simulink library "sm_excv_underc_lib"  (R2023b)
settings: Solver=VariableStepAuto  StartTime=0.0  StopTime=10.0  RelTol=1e-3
undefined symbols (not defined in the file): Excv, L1, L2, L3, L4, L5, L6, L7, L8, L9, P1, P2, P3, P4, P5, P6, P7, P8, P9, shoe_w, X, Y, Z
libraries: sm_tracked_vehicle_lib x70, sm_lib x54, nesl_utility x32, sm_excv_scene_lib x9, fl_lib x8, sm_excv_frame_lib x4
(part 4 of 5)

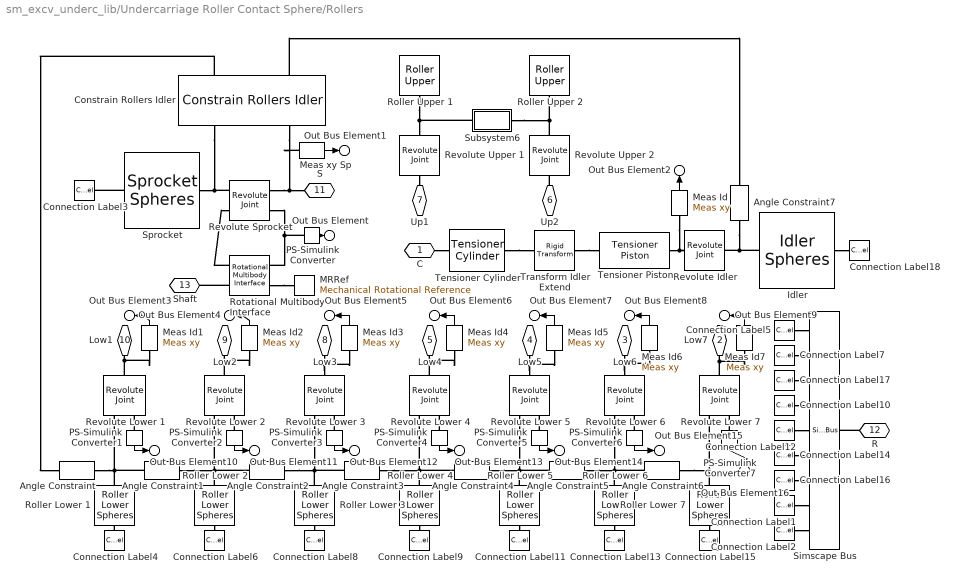
== system sm_excv_underc_lib/Undercarriage Roller Contact Sphere/Rollers ==
  Angle Constraint{,1..7} (8 alike) : sm_tracked_vehicle_lib/Angle Constraint  SystemSampleTime=-1  VariantActivationTime=update diagram  AllowFlexibleInterface=on  Latency=0  AutoFrameSizeCalculation=off
  Connection Label1 : ConnectionLabel  Label=Spr
  Connection Label10 : ConnectionLabel  Label=L4
  Connection Label11 : ConnectionLabel  Label=L5
  Connection Label12 : ConnectionLabel  Label=L5
  Connection Label13 : ConnectionLabel  Label=L6
  Connection Label14 : ConnectionLabel  Label=L6
  Connection Label15 : ConnectionLabel  Label=L7
  Connection Label16 : ConnectionLabel  Label=L7
  Connection Label17 : ConnectionLabel  Label=L3
  Connection Label18 : ConnectionLabel  Label=Idl
  Connection Label2 : ConnectionLabel  Label=Idl
  Connection Label3 : ConnectionLabel  Label=Spr
  Connection Label4 : ConnectionLabel  Label=L1
  Connection Label5 : ConnectionLabel  Label=L1
  Connection Label6 : ConnectionLabel  Label=L2
  Connection Label7 : ConnectionLabel  Label=L2
  Connection Label8 : ConnectionLabel  Label=L3
  Connection Label9 : ConnectionLabel  Label=L4
  Constrain Rollers Idler : sm_tracked_vehicle_lib/Constrain Rollers Idler  sprk_rolling_rad=sprk_rolling_rad  roller_lower_rolling_rad=roller_lower_rolling_rad  idler_rolling_rad=idler_rolling_rad
  Idler : sm_tracked_vehicle_lib/Idler Spheres  idler_rad=idler_rad  idler_len=idler_len  idler_rho=idler_rho  idler_clr=idler_clr  idler_opc=idler_opc  idler_rolling_rad=idler_rolling_rad  idler_contact_geo_width=shoe_w  idler_contact_geo_clr=idler_contact_geo_clr  idler_contact_geo_opc=idler_contact_geo_opc
  MRRef : fl_lib/Mechanical/Rotational Elements/Mechanical Rotational Reference
  Meas Id{,1..7} (8 alike) : sm_excv_scene_lib/Meas xy  whl_offset=Excv.Shoe.w
  Meas xy Sp : sm_excv_scene_lib/Meas xy  whl_offset=Excv.Shoe.w
  PS-Simulink Converter{,1..7} (8 alike) : nesl_utility/PS-Simulink Converter  PhysicalDomain=network_engine_domain  SubClassName=ps_output  LeftPortType=input  RightPortType=output  PseudoPeriodic=off  Frequencies=[]  VectorFormat=inherit  Unit=inherit  AffineConversion=off
  Revolute Idler : sm_lib/Joints/Revolute Joint  JointMode=Normal  SenseConstraintForce=off  SenseConstraintForceX=off  SenseConstraintForceY=off  SenseConstraintForceZ=off  SenseConstraintTorque=off  SenseConstraintTorqueX=off  SenseConstraintTorqueY=off  SenseConstraintTorqueZ=off  SenseTotalForce=off  SenseTotalForceX=off  SenseTotalForceY=off  SenseTotalForceZ=off  SenseTotalTorque=off  SenseTotalTorqueX=off  SenseTotalTorqueY=off  SenseTotalTorqueZ=off  CompositeWrenchDir=FollowerOnBase  CompositeWrenchFrame=BaseFrame  EquilibriumPosition=0  EquilibriumPositionUnits=rad  SpringStiffness=0  SpringStiffnessUnits=N*m/rad  DampingCoefficient=0  DampingCoefficientUnits=N*m/(rad/s)  TorqueActuationMode=NoTorque  MotionActuationMode=ComputedMotion  SensePosition=off  SenseVelocity=off  SenseAcceleration=off  SenseTorqueForce=off  SenseLowerLimitTorqueForce=off  SenseUpperLimitTorqueForce=off  LowerLimitSpecify=off  LowerLimitBound=-90  LowerLimitBoundUnits=deg  LowerLimitStiffness=1e4  LowerLimitStiffnessUnits=N*m/deg  LowerLimitDamping=10  LowerLimitDampingUnits=N*m/(deg/s)  LowerLimitTransitionRegionWidth=0.1  LowerLimitTransitionRegionWidthUnits=deg  UpperLimitSpecify=off  UpperLimitBound=90  UpperLimitBoundUnits=deg  UpperLimitStiffness=1e4  UpperLimitStiffnessUnits=N*m/deg  UpperLimitDamping=10  UpperLimitDampingUnits=N*m/(deg/s)  UpperLimitTransitionRegionWidth=0.1  UpperLimitTransitionRegionWidthUnits=deg  PositionTargetSpecify=off  PositionTargetPriority=Low  PositionTargetValue=0  PositionTargetValueUnits=deg  VelocityTargetSpecify=off  VelocityTargetPriority=High  VelocityTargetValue=0  VelocityTargetValueUnits=deg/s
  Revolute Lower {1..7} (7 alike) : sm_lib/Joints/Revolute Joint  JointMode=Normal  SenseConstraintForce=off  SenseConstraintForceX=off  SenseConstraintForceY=off  SenseConstraintForceZ=off  SenseConstraintTorque=off  SenseConstraintTorqueX=off  SenseConstraintTorqueY=off  SenseConstraintTorqueZ=off  SenseTotalForce=off  SenseTotalForceX=off  SenseTotalForceY=off  SenseTotalForceZ=off  SenseTotalTorque=off  SenseTotalTorqueX=off  SenseTotalTorqueY=off  SenseTotalTorqueZ=off  CompositeWrenchDir=FollowerOnBase  CompositeWrenchFrame=BaseFrame  EquilibriumPosition=0  EquilibriumPositionUnits=rad  SpringStiffness=0  SpringStiffnessUnits=N*m/rad  DampingCoefficient=0  DampingCoefficientUnits=N*m/(rad/s)  TorqueActuationMode=NoTorque  MotionActuationMode=ComputedMotion  SensePosition=off  SenseVelocity=off  SenseAcceleration=off  SenseTorqueForce=on  SenseLowerLimitTorqueForce=off  SenseUpperLimitTorqueForce=off  LowerLimitSpecify=off  LowerLimitBound=-90  LowerLimitBoundUnits=deg  LowerLimitStiffness=1e4  LowerLimitStiffnessUnits=N*m/deg  LowerLimitDamping=10  LowerLimitDampingUnits=N*m/(deg/s)  LowerLimitTransitionRegionWidth=0.1  LowerLimitTransitionRegionWidthUnits=deg  UpperLimitSpecify=off  UpperLimitBound=90  UpperLimitBoundUnits=deg  UpperLimitStiffness=1e4  UpperLimitStiffnessUnits=N*m/deg  UpperLimitDamping=10  UpperLimitDampingUnits=N*m/(deg/s)  UpperLimitTransitionRegionWidth=0.1  UpperLimitTransitionRegionWidthUnits=deg  PositionTargetSpecify=off  PositionTargetPriority=Low  PositionTargetValue=0  PositionTargetValueUnits=deg  VelocityTargetSpecify=off  VelocityTargetPriority=High  VelocityTargetValue=0  VelocityTargetValueUnits=deg/s
  Revolute Sprocket : sm_lib/Joints/Revolute Joint  JointMode=Normal  SenseConstraintForce=off  SenseConstraintForceX=off  SenseConstraintForceY=off  SenseConstraintForceZ=off  SenseConstraintTorque=off  SenseConstraintTorqueX=off  SenseConstraintTorqueY=off  SenseConstraintTorqueZ=off  SenseTotalForce=off  SenseTotalForceX=off  SenseTotalForceY=off  SenseTotalForceZ=off  SenseTotalTorque=off  SenseTotalTorqueX=off  SenseTotalTorqueY=off  SenseTotalTorqueZ=off  CompositeWrenchDir=FollowerOnBase  CompositeWrenchFrame=BaseFrame  EquilibriumPosition=0  EquilibriumPositionUnits=rad  SpringStiffness=0  SpringStiffnessUnits=N*m/rad  DampingCoefficient=0  DampingCoefficientUnits=N*m/(rad/s)  TorqueActuationMode=InputTorque  MotionActuationMode=ComputedMotion  SensePosition=off  SenseVelocity=on  SenseAcceleration=off  SenseTorqueForce=off  SenseLowerLimitTorqueForce=off  SenseUpperLimitTorqueForce=off  LowerLimitSpecify=off  LowerLimitBound=-90  LowerLimitBoundUnits=deg  LowerLimitStiffness=1e4  LowerLimitStiffnessUnits=N*m/deg  LowerLimitDamping=10  LowerLimitDampingUnits=N*m/(deg/s)  LowerLimitTransitionRegionWidth=0.1  LowerLimitTransitionRegionWidthUnits=deg  UpperLimitSpecify=off  UpperLimitBound=90  UpperLimitBoundUnits=deg  UpperLimitStiffness=1e4  UpperLimitStiffnessUnits=N*m/deg  UpperLimitDamping=10  UpperLimitDampingUnits=N*m/(deg/s)  UpperLimitTransitionRegionWidth=0.1  UpperLimitTransitionRegionWidthUnits=deg  PositionTargetSpecify=off  PositionTargetPriority=Low  PositionTargetValue=0  PositionTargetValueUnits=deg  VelocityTargetSpecify=off  VelocityTargetPriority=High  VelocityTargetValue=0  VelocityTargetValueUnits=deg/s
  Revolute Upper 1 : sm_lib/Joints/Revolute Joint  JointMode=Normal  SenseConstraintForce=off  SenseConstraintForceX=off  SenseConstraintForceY=off  SenseConstraintForceZ=off  SenseConstraintTorque=off  SenseConstraintTorqueX=off  SenseConstraintTorqueY=off  SenseConstraintTorqueZ=off  SenseTotalForce=off  SenseTotalForceX=off  SenseTotalForceY=off  SenseTotalForceZ=off  SenseTotalTorque=off  SenseTotalTorqueX=off  SenseTotalTorqueY=off  SenseTotalTorqueZ=off  CompositeWrenchDir=FollowerOnBase  CompositeWrenchFrame=BaseFrame  EquilibriumPosition=0  EquilibriumPositionUnits=rad  SpringStiffness=0  SpringStiffnessUnits=N*m/rad  DampingCoefficient=0  DampingCoefficientUnits=N*m/(rad/s)  TorqueActuationMode=NoTorque  MotionActuationMode=ComputedMotion  SensePosition=off  SenseVelocity=off  SenseAcceleration=off  SenseTorqueForce=off  SenseLowerLimitTorqueForce=off  SenseUpperLimitTorqueForce=off  LowerLimitSpecify=off  LowerLimitBound=-90  LowerLimitBoundUnits=deg  LowerLimitStiffness=1e4  LowerLimitStiffnessUnits=N*m/deg  LowerLimitDamping=10  LowerLimitDampingUnits=N*m/(deg/s)  LowerLimitTransitionRegionWidth=0.1  LowerLimitTransitionRegionWidthUnits=deg  UpperLimitSpecify=off  UpperLimitBound=90  UpperLimitBoundUnits=deg  UpperLimitStiffness=1e4  UpperLimitStiffnessUnits=N*m/deg  UpperLimitDamping=10  UpperLimitDampingUnits=N*m/(deg/s)  UpperLimitTransitionRegionWidth=0.1  UpperLimitTransitionRegionWidthUnits=deg  PositionTargetSpecify=off  PositionTargetPriority=Low  PositionTargetValue=0  PositionTargetValueUnits=deg  VelocityTargetSpecify=off  VelocityTargetPriority=High  VelocityTargetValue=0  VelocityTargetValueUnits=deg/s
  Revolute Upper 2 : sm_lib/Joints/Revolute Joint  JointMode=Normal  SenseConstraintForce=off  SenseConstraintForceX=off  SenseConstraintForceY=off  SenseConstraintForceZ=off  SenseConstraintTorque=off  SenseConstraintTorqueX=off  SenseConstraintTorqueY=off  SenseConstraintTorqueZ=off  SenseTotalForce=off  SenseTotalForceX=off  SenseTotalForceY=off  SenseTotalForceZ=off  SenseTotalTorque=off  SenseTotalTorqueX=off  SenseTotalTorqueY=off  SenseTotalTorqueZ=off  CompositeWrenchDir=FollowerOnBase  CompositeWrenchFrame=BaseFrame  EquilibriumPosition=0  EquilibriumPositionUnits=rad  SpringStiffness=0  SpringStiffnessUnits=N*m/rad  DampingCoefficient=0  DampingCoefficientUnits=N*m/(rad/s)  TorqueActuationMode=NoTorque  MotionActuationMode=ComputedMotion  SensePosition=off  SenseVelocity=off  SenseAcceleration=off  SenseTorqueForce=off  SenseLowerLimitTorqueForce=off  SenseUpperLimitTorqueForce=off  LowerLimitSpecify=off  LowerLimitBound=-90  LowerLimitBoundUnits=deg  LowerLimitStiffness=1e4  LowerLimitStiffnessUnits=N*m/deg  LowerLimitDamping=10  LowerLimitDampingUnits=N*m/(deg/s)  LowerLimitTransitionRegionWidth=0.1  LowerLimitTransitionRegionWidthUnits=deg  UpperLimitSpecify=off  UpperLimitBound=90  UpperLimitBoundUnits=deg  UpperLimitStiffness=1e4  UpperLimitStiffnessUnits=N*m/deg  UpperLimitDamping=10  UpperLimitDampingUnits=N*m/(deg/s)  UpperLimitTransitionRegionWidth=0.1  UpperLimitTransitionRegionWidthUnits=deg  PositionTargetSpecify=off  PositionTargetPriority=Low  PositionTargetValue=0  PositionTargetValueUnits=deg  VelocityTargetSpecify=off  VelocityTargetPriority=High  VelocityTargetValue=0  VelocityTargetValueUnits=deg/s
  Roller Lower {1..7} (7 alike) : sm_tracked_vehicle_lib/Roller Lower Spheres  roller_lower_rad=roller_lower_rad  roller_lower_len=roller_lower_len  roller_lower_rho=roller_lower_rho  roller_lower_clr=roller_lower_clr  roller_lower_opc=roller_lower_opc  roller_lower_rolling_rad=roller_lower_rolling_rad  roller_lower_contgeo_width=shoe_w  roller_lower_contgeo_clr=roller_lower_contgeo_clr  roller_lower_contgeo_opc=roller_lower_contgeo_opc
      settings: LibrarySourceBlock=sm_chain_drive_lib/Pulley_Bot
  Roller Upper 1 : sm_tracked_vehicle_lib/Roller Upper  roller_upper_rad=roller_upper_rad  roller_upper_len=roller_upper_len  roller_upper_rho=roller_upper_rho  roller_upper_clr=roller_upper_clr  roller_upper_opc=roller_upper_opc  roller_upper_contgeo_clr=roller_upper_contgeo_clr  roller_upper_contgeo_opc=roller_upper_contgeo_opc
      settings: LibrarySourceBlock=sm_chain_drive_lib/Pulley_Top
  Roller Upper 2 : sm_tracked_vehicle_lib/Roller Upper  roller_upper_rad=roller_upper_rad  roller_upper_len=roller_upper_len  roller_upper_rho=roller_upper_rho  roller_upper_clr=roller_upper_clr  roller_upper_opc=roller_upper_opc  roller_upper_contgeo_clr=roller_upper_contgeo_clr  roller_upper_contgeo_opc=roller_upper_contgeo_opc
      settings: LibrarySourceBlock=sm_chain_drive_lib/Pulley_Top
  Rotational Multibody Interface : fl_lib/Mechanical/Multibody Interfaces/Rotational Multibody Interface
  Simscape Bus : SimscapeBus  HierarchyStrings=L1;L2;L3;L4;L5;L6;L7;L8;L9
  Sprocket : sm_tracked_vehicle_lib/Sprocket Spheres  sprk_xc=sprk_xc  sprk_len=sprk_len  sprk_rho=sprk_rho  sprk_clr=sprk_clr  sprk_opc=sprk_opc  sprk_rolling_rad=sprk_rolling_rad  sprk_contact_geo_w=shoe_w  sprk_contact_geo_clr=sprk_contact_geo_clr  sprk_contact_geo_opc=sprk_contact_geo_opc
  Subsystem6 : Subsystem
  Tensioner Cylinder : sm_tracked_vehicle_lib/Tensioner Cylinder  cyl_rad=tensioner_cyl_rad  cyl_len=tensioner_cyl_len  cyl_rho=tensioner_cyl_rho  cyl_clr=tensioner_cyl_clr  cyl_opc=tensioner_cyl_opc
      settings: LibrarySourceBlock=sm_chain_drive_lib/Idler_Housing
  Tensioner Piston : sm_tracked_vehicle_lib/Tensioner Piston  pist_rad=tensioner_pist_rad  pist_len=tensioner_pist_len  pist_rho=tensioner_pist_rho  pist_clr=tensioner_pist_clr  pist_opc=tensioner_pist_opc  br_height=tensioner_br_height  br_length=tensioner_br_length  br_width=tensioner_br_width  br_rho=tensioner_br_rho  br_thk=tensioner_br_thk  br_clr=tensioner_br_clr  br_opc=tensioner_br_opc
      settings: LibrarySourceBlock=sm_chain_drive_lib/ldler_Damper
  Transform Idler Extend : sm_lib/Frames and Transforms/Rigid Transform  TranslationMethod=StandardAxis  TranslationStandardOffset=idler_max_ext  TranslationStandardOffsetUnits=m  TranslationStandardAxis=+Z  TranslationCartesianOffset=[0 0 0]  TranslationCartesianOffsetUnits=m  TranslationROffset=0  TranslationROffsetUnits=m  TranslationZOffset=0  TranslationZOffsetUnits=m  TranslationThetaOffset=0  TranslationThetaOffsetUnits=deg  RotationMethod=None  RotationAngleUnits=deg  RotationStandardAxis=+Z  RotationAngle=0.1  RotationArbitraryAxis=[0 0 1]  FollAlignAxisA=+X  BaseAlignAxisA=+Y  FollAlignAxisB=+Y  BaseAlignAxisB=+Z  RotationSequenceAxes=FollowerAxes  RotationSequence=XYX  RotationSequenceAngles=[0 0 0]  RotationSequenceAnglesUnits=deg  RotationMatrix=[1 0 0; 0 1 0; 0 0 1]  Quaternion=[1 0 0 0]
  C : PMIOPort  Side=Left
  Low7 : PMIOPort  Port=2  Side=Left
  Low6 : PMIOPort  Port=3  Side=Left
  Low5 : PMIOPort  Port=4  Side=Left
  Low4 : PMIOPort  Port=5  Side=Left
  Up2 : PMIOPort  Port=6  Side=Left
  Up1 : PMIOPort  Port=7  Side=Left
  Low3 : PMIOPort  Port=8  Side=Left
  Low2 : PMIOPort  Port=9  Side=Left
  Low1 : PMIOPort  Port=10  Side=Left
  S : PMIOPort  Port=11  Side=Left
  R : PMIOPort  Port=12  Side=Right
  Shaft : PMIOPort  Port=13  Side=Right
  Out Bus Element : Outport  PortName=m  Element=tSprk
  Out Bus Element1 : Outport  PortName=m  Element=Sp
  Out Bus Element2 : Outport  PortName=m  Element=Id
  Out Bus Element3 : Outport  PortName=m  Element=LR1
  Out Bus Element4 : Outport  PortName=m  Element=LR2
  Out Bus Element5 : Outport  PortName=m  Element=LR3
  Out Bus Element6 : Outport  PortName=m  Element=LR4
  Out Bus Element7 : Outport  PortName=m  Element=LR5
  Out Bus Element8 : Outport  PortName=m  Element=LR6
  Out Bus Element9 : Outport  PortName=m  Element=LR7
  Out Bus Element10 : Outport  PortName=m  Element=RL1
  Out Bus Element11 : Outport  PortName=m  Element=RL2
  Out Bus Element12 : Outport  PortName=m  Element=RL3
  Out Bus Element13 : Outport  PortName=m  Element=RL4
  Out Bus Element14 : Outport  PortName=m  Element=RL5
  Out Bus Element15 : Outport  PortName=m  Element=RL6
  Out Bus Element16 : Outport  PortName=m  Element=RL7
  wires:
  PS-Simulink Converter/1 -> Out Bus Element/1
  Meas xy Sp/1 -> Out Bus Element1/1
  Meas Id/1 -> Out Bus Element2/1
  Meas Id1/1 -> Out Bus Element3/1
  Meas Id2/1 -> Out Bus Element4/1
  Meas Id3/1 -> Out Bus Element5/1
  Meas Id4/1 -> Out Bus Element6/1
  Meas Id5/1 -> Out Bus Element7/1
  Meas Id6/1 -> Out Bus Element8/1
  Meas Id7/1 -> Out Bus Element9/1
  PS-Simulink Converter1/1 -> Out Bus Element10/1
  PS-Simulink Converter6/1 -> Out Bus Element15/1
  PS-Simulink Converter4/1 -> Out Bus Element13/1
  PS-Simulink Converter3/1 -> Out Bus Element12/1
  PS-Simulink Converter5/1 -> Out Bus Element14/1
  PS-Simulink Converter2/1 -> Out Bus Element11/1
  PS-Simulink Converter7/1 -> Out Bus Element16/1
  connections:
  Connection Label2/LConn1 -- Simscape Bus/LConn9
  Constrain Rollers Idler/RConn1 -- Angle Constraint/LConn1
  Constrain Rollers Idler/RConn2 -- Angle Constraint7/LConn1
  Tensioner Cylinder/RConn1 -- Transform Idler Extend/LConn1
  C/RConn1 -- Tensioner Cylinder/LConn1
  Transform Idler Extend/RConn1 -- Tensioner Piston/LConn1
  Idler/RConn1 -- Connection Label18/LConn1
  Revolute Upper 1/LConn1 -- Up1/RConn1
  Angle Constraint5/RConn1 -- Revolute Lower 6/RConn1 -- Roller Lower 6/LConn1 -- Angle Constraint6/LConn1
  S/RConn1 -- Meas xy Sp/LConn1 -- Constrain Rollers Idler/LConn2 -- Revolute Sprocket/LConn1
  R/RConn1 -- Simscape Bus/RConn1
  Revolute Idler/RConn1 -- Idler/LConn1 -- Angle Constraint7/RConn1
  Sprocket/LConn1 -- Constrain Rollers Idler/LConn1 -- Revolute Sprocket/RConn1
  Angle Constraint4/RConn1 -- Revolute Lower 5/RConn1 -- Roller Lower 5/LConn1 -- Angle Constraint5/LConn1
  Subsystem6/RConn1 -- Roller Upper 2/LConn1 -- Revolute Upper 2/RConn1
  Revolute Lower 2/LConn1 -- Meas Id2/LConn1 -- Low2/RConn1
  Tensioner Piston/RConn1 -- Meas Id/LConn1 -- Revolute Idler/LConn1
  Sprocket/RConn1 -- Connection Label3/LConn1
  Connection Label4/LConn1 -- Roller Lower 1/RConn1
  Revolute Lower 4/LConn1 -- Meas Id4/LConn1 -- Low4/RConn1
  Angle Constraint2/RConn1 -- Revolute Lower 3/RConn1 -- Roller Lower 3/LConn1 -- Angle Constraint3/LConn1
  Revolute Lower 7/LConn1 -- Meas Id7/LConn1 -- Low7/RConn1
  Revolute Lower 1/LConn1 -- Low1/RConn1 -- Meas Id1/LConn1
  Connection Label10/LConn1 -- Simscape Bus/LConn4
  Connection Label17/LConn1 -- Simscape Bus/LConn3
  Connection Label16/LConn1 -- Simscape Bus/LConn7
  Connection Label14/LConn1 -- Simscape Bus/LConn6
  Connection Label12/LConn1 -- Simscape Bus/LConn5
  Connection Label5/LConn1 -- Simscape Bus/LConn1
  Low5/RConn1 -- Meas Id5/LConn1 -- Revolute Lower 5/LConn1
  Angle Constraint2/LConn1 -- Revolute Lower 2/RConn1 -- Angle Constraint1/RConn1 -- Roller Lower 2/LConn1
  Low3/RConn1 -- Meas Id3/LConn1 -- Revolute Lower 3/LConn1
  Angle Constraint6/RConn1 -- Revolute Lower 7/RConn1 -- Roller Lower 7/LConn1
  Angle Constraint1/LConn1 -- Roller Lower 1/LConn1 -- Angle Constraint/RConn1 -- Revolute Lower 1/RConn1
  Angle Constraint4/LConn1 -- Revolute Lower 4/RConn1 -- Angle Constraint3/RConn1 -- Roller Lower 4/LConn1
  Low6/RConn1 -- Meas Id6/LConn1 -- Revolute Lower 6/LConn1
  Revolute Upper 1/RConn1 -- Subsystem6/LConn1 -- Roller Upper 1/LConn1
  Up2/RConn1 -- Revolute Upper 2/LConn1
  Revolute Sprocket/LConn2 -- Rotational Multibody Interface/LConn1 -- PS-Simulink Converter/LConn1
  Rotational Multibody Interface/RConn1 -- Revolute Sprocket/RConn2
  Rotational Multibody Interface/RConn2 -- Shaft/RConn1
  Rotational Multibody Interface/LConn2 -- MRRef/LConn1
  Roller Lower 2/RConn1 -- Connection Label6/LConn1
  Roller Lower 3/RConn1 -- Connection Label8/LConn1
  Roller Lower 4/RConn1 -- Connection Label9/LConn1
  Roller Lower 5/RConn1 -- Connection Label11/LConn1
  Roller Lower 6/RConn1 -- Connection Label13/LConn1
  Roller Lower 7/RConn1 -- Connection Label15/LConn1
  Connection Label7/LConn1 -- Simscape Bus/LConn2
  Connection Label1/LConn1 -- Simscape Bus/LConn8
  PS-Simulink Converter1/LConn1 -- Revolute Lower 1/RConn2
  PS-Simulink Converter2/LConn1 -- Revolute Lower 2/RConn2
  PS-Simulink Converter3/LConn1 -- Revolute Lower 3/RConn2
  PS-Simulink Converter4/LConn1 -- Revolute Lower 4/RConn2
  PS-Simulink Converter5/LConn1 -- Revolute Lower 5/RConn2
  PS-Simulink Converter6/LConn1 -- Revolute Lower 6/RConn2
  PS-Simulink Converter7/LConn1 -- Revolute Lower 7/RConn2

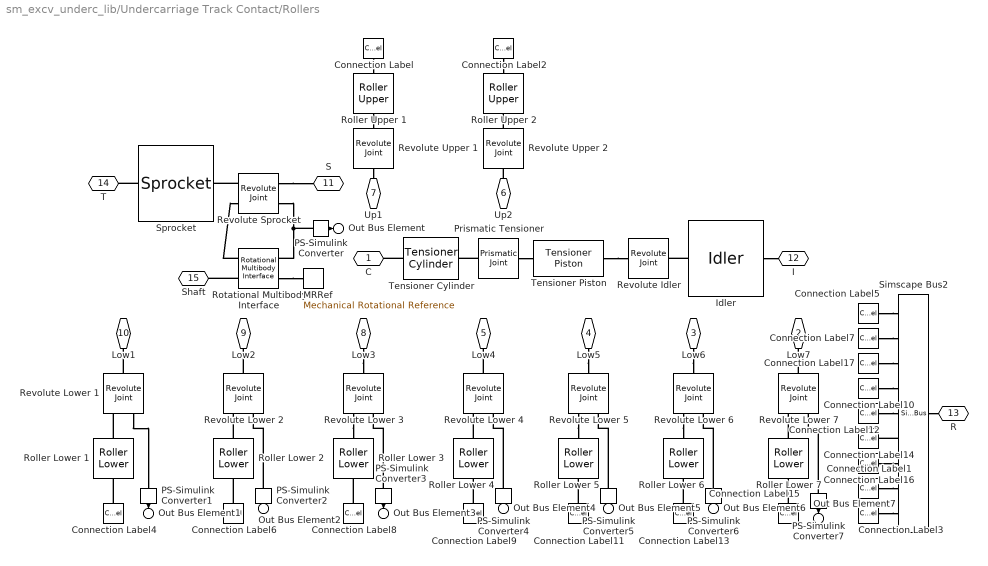
== system sm_excv_underc_lib/Undercarriage Track Contact/Rollers ==
  Connection Label : ConnectionLabel  Label=U1
  Connection Label1 : ConnectionLabel  Label=U1
  Connection Label10 : ConnectionLabel  Label=L4
  Connection Label11 : ConnectionLabel  Label=L5
  Connection Label12 : ConnectionLabel  Label=L5
  Connection Label13 : ConnectionLabel  Label=L6
  Connection Label14 : ConnectionLabel  Label=L6
  Connection Label15 : ConnectionLabel  Label=L7
  Connection Label16 : ConnectionLabel  Label=L7
  Connection Label17 : ConnectionLabel  Label=L3
  Connection Label2 : ConnectionLabel  Label=U2
  Connection Label3 : ConnectionLabel  Label=U2
  Connection Label4 : ConnectionLabel  Label=L1
  Connection Label5 : ConnectionLabel  Label=L1
  Connection Label6 : ConnectionLabel  Label=L2
  Connection Label7 : ConnectionLabel  Label=L2
  Connection Label8 : ConnectionLabel  Label=L3
  Connection Label9 : ConnectionLabel  Label=L4
  Idler : sm_tracked_vehicle_lib/Idler  idler_rad=idler_rad  idler_len=idler_len  idler_rho=idler_rho  idler_clr=idler_clr  idler_opc=idler_opc  idler_contgeo_clr=idler_contgeo_clr  idler_contgeo_opc=idler_contgeo_opc
  MRRef : fl_lib/Mechanical/Rotational Elements/Mechanical Rotational Reference
  PS-Simulink Converter{,1..7} (8 alike) : nesl_utility/PS-Simulink Converter  PhysicalDomain=network_engine_domain  SubClassName=ps_output  LeftPortType=input  RightPortType=output  PseudoPeriodic=off  Frequencies=[]  VectorFormat=inherit  Unit=inherit  AffineConversion=off
  Prismatic Tensioner : sm_lib/Joints/Prismatic Joint  JointMode=Normal  SenseConstraintForce=off  SenseConstraintForceX=off  SenseConstraintForceY=off  SenseConstraintForceZ=off  SenseConstraintTorque=off  SenseConstraintTorqueX=off  SenseConstraintTorqueY=off  SenseConstraintTorqueZ=off  SenseTotalForce=off  SenseTotalForceX=off  SenseTotalForceY=off  SenseTotalForceZ=off  SenseTotalTorque=off  SenseTotalTorqueX=off  SenseTotalTorqueY=off  SenseTotalTorqueZ=off  CompositeWrenchDir=FollowerOnBase  CompositeWrenchFrame=BaseFrame  EquilibriumPosition=tensioner_eqpos  EquilibriumPositionUnits=m  SpringStiffness=tensioner_k  SpringStiffnessUnits=N/m  DampingCoefficient=tensioner_b  DampingCoefficientUnits=N/(m/s)  TorqueActuationMode=NoTorque  MotionActuationMode=ComputedMotion  SensePosition=off  SenseVelocity=off  SenseAcceleration=off  SenseTorqueForce=off  SenseLowerLimitTorqueForce=off  SenseUpperLimitTorqueForce=off  LowerLimitSpecify=off  LowerLimitBound=-1  LowerLimitBoundUnits=m  LowerLimitStiffness=1e6  LowerLimitStiffnessUnits=N/m  LowerLimitDamping=1e3  LowerLimitDampingUnits=N/(m/s)  LowerLimitTransitionRegionWidth=1e-4  LowerLimitTransitionRegionWidthUnits=m  UpperLimitSpecify=off  UpperLimitBound=1  UpperLimitBoundUnits=m  UpperLimitStiffness=1e6  UpperLimitStiffnessUnits=N/m  UpperLimitDamping=1e3  UpperLimitDampingUnits=N/(m/s)  UpperLimitTransitionRegionWidth=1e-4  UpperLimitTransitionRegionWidthUnits=m  PositionTargetSpecify=on  PositionTargetPriority=High  PositionTargetValue=tensioner_x0  PositionTargetValueUnits=m  VelocityTargetSpecify=off  VelocityTargetPriority=High  VelocityTargetValue=0  VelocityTargetValueUnits=m/s
  Revolute Idler : sm_lib/Joints/Revolute Joint  JointMode=Normal  SenseConstraintForce=off  SenseConstraintForceX=off  SenseConstraintForceY=off  SenseConstraintForceZ=off  SenseConstraintTorque=off  SenseConstraintTorqueX=off  SenseConstraintTorqueY=off  SenseConstraintTorqueZ=off  SenseTotalForce=off  SenseTotalForceX=off  SenseTotalForceY=off  SenseTotalForceZ=off  SenseTotalTorque=off  SenseTotalTorqueX=off  SenseTotalTorqueY=off  SenseTotalTorqueZ=off  CompositeWrenchDir=FollowerOnBase  CompositeWrenchFrame=BaseFrame  EquilibriumPosition=0  EquilibriumPositionUnits=rad  SpringStiffness=0  SpringStiffnessUnits=N*m/rad  DampingCoefficient=0  DampingCoefficientUnits=N*m/(rad/s)  TorqueActuationMode=NoTorque  MotionActuationMode=ComputedMotion  SensePosition=off  SenseVelocity=off  SenseAcceleration=off  SenseTorqueForce=off  SenseLowerLimitTorqueForce=off  SenseUpperLimitTorqueForce=off  LowerLimitSpecify=off  LowerLimitBound=-90  LowerLimitBoundUnits=deg  LowerLimitStiffness=1e4  LowerLimitStiffnessUnits=N*m/deg  LowerLimitDamping=10  LowerLimitDampingUnits=N*m/(deg/s)  LowerLimitTransitionRegionWidth=0.1  LowerLimitTransitionRegionWidthUnits=deg  UpperLimitSpecify=off  UpperLimitBound=90  UpperLimitBoundUnits=deg  UpperLimitStiffness=1e4  UpperLimitStiffnessUnits=N*m/deg  UpperLimitDamping=10  UpperLimitDampingUnits=N*m/(deg/s)  UpperLimitTransitionRegionWidth=0.1  UpperLimitTransitionRegionWidthUnits=deg  PositionTargetSpecify=off  PositionTargetPriority=Low  PositionTargetValue=0  PositionTargetValueUnits=deg  VelocityTargetSpecify=off  VelocityTargetPriority=High  VelocityTargetValue=0  VelocityTargetValueUnits=deg/s
  Revolute Lower {1..7} (7 alike) : sm_lib/Joints/Revolute Joint  JointMode=Normal  SenseConstraintForce=off  SenseConstraintForceX=off  SenseConstraintForceY=off  SenseConstraintForceZ=off  SenseConstraintTorque=off  SenseConstraintTorqueX=off  SenseConstraintTorqueY=off  SenseConstraintTorqueZ=off  SenseTotalForce=off  SenseTotalForceX=off  SenseTotalForceY=off  SenseTotalForceZ=off  SenseTotalTorque=off  SenseTotalTorqueX=off  SenseTotalTorqueY=off  SenseTotalTorqueZ=off  CompositeWrenchDir=FollowerOnBase  CompositeWrenchFrame=BaseFrame  EquilibriumPosition=0  EquilibriumPositionUnits=rad  SpringStiffness=0  SpringStiffnessUnits=N*m/rad  DampingCoefficient=0  DampingCoefficientUnits=N*m/(rad/s)  TorqueActuationMode=NoTorque  MotionActuationMode=ComputedMotion  SensePosition=off  SenseVelocity=off  SenseAcceleration=off  SenseTorqueForce=on  SenseLowerLimitTorqueForce=off  SenseUpperLimitTorqueForce=off  LowerLimitSpecify=off  LowerLimitBound=-90  LowerLimitBoundUnits=deg  LowerLimitStiffness=1e4  LowerLimitStiffnessUnits=N*m/deg  LowerLimitDamping=10  LowerLimitDampingUnits=N*m/(deg/s)  LowerLimitTransitionRegionWidth=0.1  LowerLimitTransitionRegionWidthUnits=deg  UpperLimitSpecify=off  UpperLimitBound=90  UpperLimitBoundUnits=deg  UpperLimitStiffness=1e4  UpperLimitStiffnessUnits=N*m/deg  UpperLimitDamping=10  UpperLimitDampingUnits=N*m/(deg/s)  UpperLimitTransitionRegionWidth=0.1  UpperLimitTransitionRegionWidthUnits=deg  PositionTargetSpecify=off  PositionTargetPriority=Low  PositionTargetValue=0  PositionTargetValueUnits=deg  VelocityTargetSpecify=off  VelocityTargetPriority=High  VelocityTargetValue=0  VelocityTargetValueUnits=deg/s
  Revolute Sprocket : sm_lib/Joints/Revolute Joint  JointMode=Normal  SenseConstraintForce=off  SenseConstraintForceX=off  SenseConstraintForceY=off  SenseConstraintForceZ=off  SenseConstraintTorque=off  SenseConstraintTorqueX=off  SenseConstraintTorqueY=off  SenseConstraintTorqueZ=off  SenseTotalForce=off  SenseTotalForceX=off  SenseTotalForceY=off  SenseTotalForceZ=off  SenseTotalTorque=off  SenseTotalTorqueX=off  SenseTotalTorqueY=off  SenseTotalTorqueZ=off  CompositeWrenchDir=FollowerOnBase  CompositeWrenchFrame=BaseFrame  EquilibriumPosition=0  EquilibriumPositionUnits=rad  SpringStiffness=0  SpringStiffnessUnits=N*m/rad  DampingCoefficient=0  DampingCoefficientUnits=N*m/(rad/s)  TorqueActuationMode=InputTorque  MotionActuationMode=ComputedMotion  SensePosition=off  SenseVelocity=on  SenseAcceleration=off  SenseTorqueForce=off  SenseLowerLimitTorqueForce=off  SenseUpperLimitTorqueForce=off  LowerLimitSpecify=off  LowerLimitBound=-90  LowerLimitBoundUnits=deg  LowerLimitStiffness=1e4  LowerLimitStiffnessUnits=N*m/deg  LowerLimitDamping=10  LowerLimitDampingUnits=N*m/(deg/s)  LowerLimitTransitionRegionWidth=0.1  LowerLimitTransitionRegionWidthUnits=deg  UpperLimitSpecify=off  UpperLimitBound=90  UpperLimitBoundUnits=deg  UpperLimitStiffness=1e4  UpperLimitStiffnessUnits=N*m/deg  UpperLimitDamping=10  UpperLimitDampingUnits=N*m/(deg/s)  UpperLimitTransitionRegionWidth=0.1  UpperLimitTransitionRegionWidthUnits=deg  PositionTargetSpecify=off  PositionTargetPriority=Low  PositionTargetValue=0  PositionTargetValueUnits=deg  VelocityTargetSpecify=off  VelocityTargetPriority=High  VelocityTargetValue=0  VelocityTargetValueUnits=deg/s
  Revolute Upper 1 : sm_lib/Joints/Revolute Joint  JointMode=Normal  SenseConstraintForce=off  SenseConstraintForceX=off  SenseConstraintForceY=off  SenseConstraintForceZ=off  SenseConstraintTorque=off  SenseConstraintTorqueX=off  SenseConstraintTorqueY=off  SenseConstraintTorqueZ=off  SenseTotalForce=off  SenseTotalForceX=off  SenseTotalForceY=off  SenseTotalForceZ=off  SenseTotalTorque=off  SenseTotalTorqueX=off  SenseTotalTorqueY=off  SenseTotalTorqueZ=off  CompositeWrenchDir=FollowerOnBase  CompositeWrenchFrame=BaseFrame  EquilibriumPosition=0  EquilibriumPositionUnits=rad  SpringStiffness=0  SpringStiffnessUnits=N*m/rad  DampingCoefficient=0  DampingCoefficientUnits=N*m/(rad/s)  TorqueActuationMode=NoTorque  MotionActuationMode=ComputedMotion  SensePosition=off  SenseVelocity=off  SenseAcceleration=off  SenseTorqueForce=off  SenseLowerLimitTorqueForce=off  SenseUpperLimitTorqueForce=off  LowerLimitSpecify=off  LowerLimitBound=-90  LowerLimitBoundUnits=deg  LowerLimitStiffness=1e4  LowerLimitStiffnessUnits=N*m/deg  LowerLimitDamping=10  LowerLimitDampingUnits=N*m/(deg/s)  LowerLimitTransitionRegionWidth=0.1  LowerLimitTransitionRegionWidthUnits=deg  UpperLimitSpecify=off  UpperLimitBound=90  UpperLimitBoundUnits=deg  UpperLimitStiffness=1e4  UpperLimitStiffnessUnits=N*m/deg  UpperLimitDamping=10  UpperLimitDampingUnits=N*m/(deg/s)  UpperLimitTransitionRegionWidth=0.1  UpperLimitTransitionRegionWidthUnits=deg  PositionTargetSpecify=off  PositionTargetPriority=Low  PositionTargetValue=0  PositionTargetValueUnits=deg  VelocityTargetSpecify=off  VelocityTargetPriority=High  VelocityTargetValue=0  VelocityTargetValueUnits=deg/s
  Revolute Upper 2 : sm_lib/Joints/Revolute Joint  JointMode=Normal  SenseConstraintForce=off  SenseConstraintForceX=off  SenseConstraintForceY=off  SenseConstraintForceZ=off  SenseConstraintTorque=off  SenseConstraintTorqueX=off  SenseConstraintTorqueY=off  SenseConstraintTorqueZ=off  SenseTotalForce=off  SenseTotalForceX=off  SenseTotalForceY=off  SenseTotalForceZ=off  SenseTotalTorque=off  SenseTotalTorqueX=off  SenseTotalTorqueY=off  SenseTotalTorqueZ=off  CompositeWrenchDir=FollowerOnBase  CompositeWrenchFrame=BaseFrame  EquilibriumPosition=0  EquilibriumPositionUnits=rad  SpringStiffness=0  SpringStiffnessUnits=N*m/rad  DampingCoefficient=0  DampingCoefficientUnits=N*m/(rad/s)  TorqueActuationMode=NoTorque  MotionActuationMode=ComputedMotion  SensePosition=off  SenseVelocity=off  SenseAcceleration=off  SenseTorqueForce=off  SenseLowerLimitTorqueForce=off  SenseUpperLimitTorqueForce=off  LowerLimitSpecify=off  LowerLimitBound=-90  LowerLimitBoundUnits=deg  LowerLimitStiffness=1e4  LowerLimitStiffnessUnits=N*m/deg  LowerLimitDamping=10  LowerLimitDampingUnits=N*m/(deg/s)  LowerLimitTransitionRegionWidth=0.1  LowerLimitTransitionRegionWidthUnits=deg  UpperLimitSpecify=off  UpperLimitBound=90  UpperLimitBoundUnits=deg  UpperLimitStiffness=1e4  UpperLimitStiffnessUnits=N*m/deg  UpperLimitDamping=10  UpperLimitDampingUnits=N*m/(deg/s)  UpperLimitTransitionRegionWidth=0.1  UpperLimitTransitionRegionWidthUnits=deg  PositionTargetSpecify=off  PositionTargetPriority=Low  PositionTargetValue=0  PositionTargetValueUnits=deg  VelocityTargetSpecify=off  VelocityTargetPriority=High  VelocityTargetValue=0  VelocityTargetValueUnits=deg/s
  Roller Lower {1..7} (7 alike) : sm_tracked_vehicle_lib/Roller Lower  roller_lower_rad=roller_lower_rad  roller_lower_len=roller_lower_len  roller_lower_rho=roller_lower_rho  roller_lower_clr=roller_lower_clr  roller_lower_opc=roller_lower_opc  roller_lower_contgeo_clr=roller_lower_contgeo_clr  roller_lower_contgeo_opc=roller_lower_contgeo_opc
      settings: LibrarySourceBlock=sm_chain_drive_lib/Pulley_Bot
  Roller Upper 1 : sm_tracked_vehicle_lib/Roller Upper  roller_upper_rad=roller_upper_rad  roller_upper_len=roller_upper_len  roller_upper_rho=roller_upper_rho  roller_upper_clr=roller_upper_clr  roller_upper_opc=roller_upper_opc  roller_upper_contgeo_clr=roller_upper_contgeo_clr  roller_upper_contgeo_opc=roller_upper_contgeo_opc
      settings: LibrarySourceBlock=sm_chain_drive_lib/Pulley_Top
  Roller Upper 2 : sm_tracked_vehicle_lib/Roller Upper  roller_upper_rad=roller_upper_rad  roller_upper_len=roller_upper_len  roller_upper_rho=roller_upper_rho  roller_upper_clr=roller_upper_clr  roller_upper_opc=roller_upper_opc  roller_upper_contgeo_clr=roller_upper_contgeo_clr  roller_upper_contgeo_opc=roller_upper_contgeo_opc
      settings: LibrarySourceBlock=sm_chain_drive_lib/Pulley_Top
  Rotational Multibody Interface : fl_lib/Mechanical/Multibody Interfaces/Rotational Multibody Interface
  Simscape Bus2 : SimscapeBus  HierarchyStrings=P1;P2;P3;P4;P5;P6;P7;P8;P9  ConnectionType=Bus: Roller_CBO
  Sprocket : sm_tracked_vehicle_lib/Sprocket  sprk_xc=sprk_xc  sprk_len=sprk_len  sprk_rho=sprk_rho  sprk_clr=sprk_clr  sprk_opc=sprk_opc  sprk_contact_geo_ptcld=sprk_contact_geo_ptcld  sprk_contact_geo_rad=sprk_contact_geo_rad  sprk_contact_geo_clr=sprk_contact_geo_clr  sprk_contact_geo_opc=sprk_contact_geo_opc
  Tensioner Cylinder : sm_tracked_vehicle_lib/Tensioner Cylinder  cyl_rad=tensioner_cyl_rad  cyl_len=tensioner_cyl_len  cyl_rho=tensioner_cyl_rho  cyl_clr=tensioner_cyl_clr  cyl_opc=tensioner_cyl_opc
      settings: LibrarySourceBlock=sm_chain_drive_lib/Idler_Housing
  Tensioner Piston : sm_tracked_vehicle_lib/Tensioner Piston  pist_rad=tensioner_pist_rad  pist_len=tensioner_pist_len  pist_rho=tensioner_pist_rho  pist_clr=tensioner_pist_clr  pist_opc=tensioner_pist_opc  br_height=tensioner_br_height  br_length=tensioner_br_length  br_width=tensioner_br_width  br_rho=tensioner_br_rho  br_thk=tensioner_br_thk  br_clr=tensioner_br_clr  br_opc=tensioner_br_opc
      settings: LibrarySourceBlock=sm_chain_drive_lib/ldler_Damper
  C : PMIOPort  Side=Left
  Low7 : PMIOPort  Port=2  Side=Left
  Low6 : PMIOPort  Port=3  Side=Left
  Low5 : PMIOPort  Port=4  Side=Left
  Low4 : PMIOPort  Port=5  Side=Left
  Up2 : PMIOPort  Port=6  Side=Left
  Up1 : PMIOPort  Port=7  Side=Left
  Low3 : PMIOPort  Port=8  Side=Left
  Low2 : PMIOPort  Port=9  Side=Left
  Low1 : PMIOPort  Port=10  Side=Left
  S : PMIOPort  Port=11  Side=Left
  I : PMIOPort  Port=12  Side=Right
  R : PMIOPort  Port=13  Side=Right
  T : PMIOPort  Port=14  Side=Right
  Shaft : PMIOPort  Port=15  Side=Right
  Out Bus Element : Outport  PortName=m  Element=tSprk
  Out Bus Element1 : Outport  PortName=m  Element=RL1
  Out Bus Element2 : Outport  PortName=m  Element=RL2
  Out Bus Element3 : Outport  PortName=m  Element=RL3
  Out Bus Element4 : Outport  PortName=m  Element=RL4
  Out Bus Element5 : Outport  PortName=m  Element=RL5
  Out Bus Element6 : Outport  PortName=m  Element=RL6
  Out Bus Element7 : Outport  PortName=m  Element=RL7
  wires:
  PS-Simulink Converter7/1 -> Out Bus Element7/1
  PS-Simulink Converter6/1 -> Out Bus Element6/1
  PS-Simulink Converter5/1 -> Out Bus Element5/1
  PS-Simulink Converter4/1 -> Out Bus Element4/1
  PS-Simulink Converter3/1 -> Out Bus Element3/1
  PS-Simulink Converter2/1 -> Out Bus Element2/1
  PS-Simulink Converter1/1 -> Out Bus Element1/1
  PS-Simulink Converter/1 -> Out Bus Element/1
  connections:
  PS-Simulink Converter7/LConn1 -- Revolute Lower 7/RConn2
  PS-Simulink Converter6/LConn1 -- Revolute Lower 6/RConn2
  PS-Simulink Converter5/LConn1 -- Revolute Lower 5/RConn2
  PS-Simulink Converter4/LConn1 -- Revolute Lower 4/RConn2
  PS-Simulink Converter3/LConn1 -- Revolute Lower 3/RConn2
  PS-Simulink Converter2/LConn1 -- Revolute Lower 2/RConn2
  Revolute Lower 1/RConn2 -- PS-Simulink Converter1/LConn1
  Rotational Multibody Interface/LConn2 -- MRRef/LConn1
  Rotational Multibody Interface/RConn2 -- Shaft/RConn1
  Rotational Multibody Interface/RConn1 -- Revolute Sprocket/RConn2
  PS-Simulink Converter/LConn1 -- Rotational Multibody Interface/LConn1 -- Revolute Sprocket/LConn2
  Up2/RConn1 -- Revolute Upper 2/LConn1
  Roller Upper 1/LConn1 -- Revolute Upper 1/RConn1
  Low6/RConn1 -- Revolute Lower 6/LConn1
  Roller Lower 4/LConn1 -- Revolute Lower 4/RConn1
  Roller Lower 1/LConn1 -- Revolute Lower 1/RConn1
  Roller Lower 7/LConn1 -- Revolute Lower 7/RConn1
  Low3/RConn1 -- Revolute Lower 3/LConn1
  Roller Lower 2/LConn1 -- Revolute Lower 2/RConn1
  Low5/RConn1 -- Revolute Lower 5/LConn1
  Prismatic Tensioner/RConn1 -- Tensioner Piston/LConn1
  Tensioner Cylinder/LConn1 -- C/RConn1
  Connection Label5/LConn1 -- Simscape Bus2/LConn1
  Connection Label12/LConn1 -- Simscape Bus2/LConn5
  Simscape Bus2/LConn6 -- Connection Label14/LConn1
  Connection Label16/LConn1 -- Simscape Bus2/LConn7
  Connection Label7/LConn1 -- Simscape Bus2/LConn2
  Connection Label17/LConn1 -- Simscape Bus2/LConn3
  Connection Label10/LConn1 -- Simscape Bus2/LConn4
  Connection Label1/LConn1 -- Simscape Bus2/LConn8
  Connection Label3/LConn1 -- Simscape Bus2/LConn9
  Connection Label2/LConn1 -- Roller Upper 2/RConn1
  Revolute Lower 1/LConn1 -- Low1/RConn1
  Revolute Lower 7/LConn1 -- Low7/RConn1
  Revolute Lower 3/RConn1 -- Roller Lower 3/LConn1
  Revolute Lower 4/LConn1 -- Low4/RConn1
  Connection Label4/LConn1 -- Roller Lower 1/RConn1
  Sprocket/RConn1 -- T/RConn1
  Tensioner Piston/RConn1 -- Revolute Idler/LConn1
  Revolute Lower 2/LConn1 -- Low2/RConn1
  Revolute Upper 2/RConn1 -- Roller Upper 2/LConn1
  Revolute Lower 5/RConn1 -- Roller Lower 5/LConn1
  Prismatic Tensioner/LConn1 -- Tensioner Cylinder/RConn1
  Revolute Sprocket/RConn1 -- Sprocket/LConn1
  Idler/LConn1 -- Revolute Idler/RConn1
  Simscape Bus2/RConn1 -- R/RConn1
  Connection Label11/LConn1 -- Roller Lower 5/RConn1
  Revolute Sprocket/LConn1 -- S/RConn1
  Connection Label8/LConn1 -- Roller Lower 3/RConn1
  Revolute Lower 6/RConn1 -- Roller Lower 6/LConn1
  Connection Label15/LConn1 -- Roller Lower 7/RConn1
  Connection Label9/LConn1 -- Roller Lower 4/RConn1
  Revolute Upper 1/LConn1 -- Up1/RConn1
  Connection Label/LConn1 -- Roller Upper 1/RConn1
  Connection Label6/LConn1 -- Roller Lower 2/RConn1
  Connection Label13/LConn1 -- Roller Lower 6/RConn1
  Idler/RConn1 -- I/RConn1
